simulink library "env_estimation_lib"  (R2016b)
settings: Solver=VariableStepAuto  StartTime=0.0  StopTime=10.0  RelTol=1e-3
undefined symbols (not defined in the file or in its folder): fsw_params
libraries: gs_prediction_lib x1, mag_vec_lib x1, sgp4_lib_fsw x1, sun_vector_lib x1, time_coord_rotation_lib x1
settings Model: Creator=taylorreynolds  LastModifiedBy=taylorreynolds

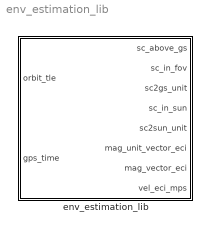
== system env_estimation_lib ==
  env_estimation_lib : Subsystem

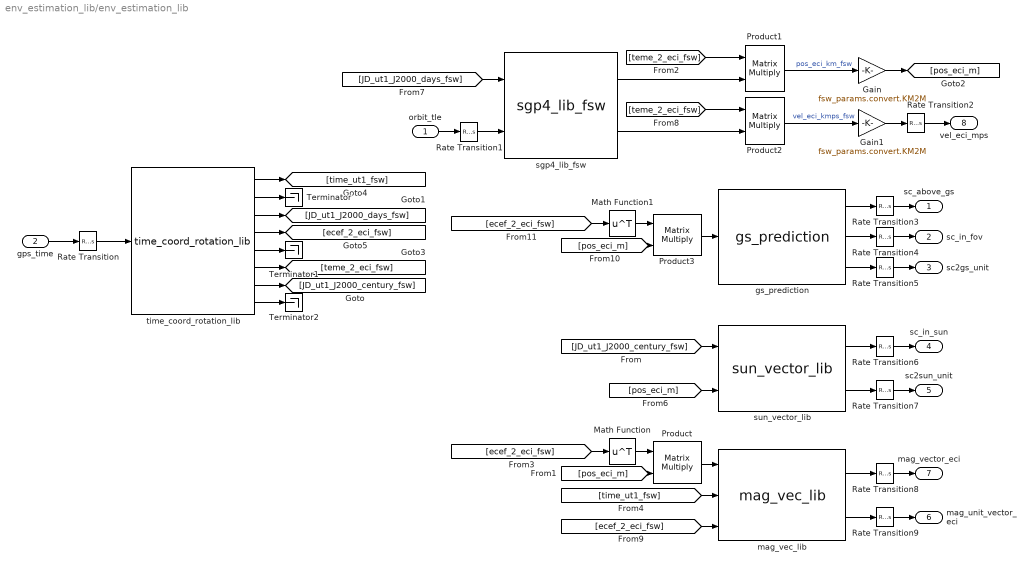
== system env_estimation_lib/env_estimation_lib ==
  orbit_tle : Inport
  gps_time : Inport  Port=2
  Gain : Gain  Gain=fsw_params.convert.KM2M
  Gain1 : Gain  Gain=fsw_params.convert.KM2M
  Math Function : Math  Operator=transpose  SaturateOnIntegerOverflow=on
  Math Function1 : Math  Operator=transpose  SaturateOnIntegerOverflow=on
  Product{,1..3} (4 alike) : Product  Multiplication=Matrix(*)
  Rate Transition : RateTransition  X0=fsw_params.env_estimation.ic.gps_time  OutPortSampleTime=fsw_params.env_estimation.sample_time_s
  Rate Transition1 : RateTransition  X0=fsw_params.env_estimation.ic.orbit_tle  OutPortSampleTime=fsw_params.env_estimation.sample_time_s
  Rate Transition{2..9} (8 alike) : RateTransition
  Terminator : Terminator
  Terminator1 : Terminator
  Terminator2 : Terminator
  gs_prediction : gs_prediction_lib/gs_prediction
  mag_vec_lib : mag_vec_lib/mag_vec_lib
  sgp4_lib_fsw : sgp4_lib_fsw/sgp4_lib_fsw
  sun_vector_lib : sun_vector_lib/sun_vector_lib
  time_coord_rotation_lib : time_coord_rotation_lib/time_coord_rotation_lib
  sc_above_gs : Outport
  sc_in_fov : Outport  Port=2
  sc2gs_unit : Outport  Port=3
  sc_in_sun : Outport  Port=4
  sc2sun_unit : Outport  Port=5
  mag_unit_vector_eci : Outport  Port=6
  mag_vector_eci : Outport  Port=7
  vel_eci_mps : Outport  Port=8
  wires:
  mag_vec_lib/2 -> Rate Transition9/1
  mag_vec_lib/1 -> Rate Transition8/1
  sun_vector_lib/2 -> Rate Transition7/1
  [teme_2_eci_fsw] -> Product1/1
  [teme_2_eci_fsw] -> Product2/1
  [ecef_2_eci_fsw] -> Math Function/1
  [JD_ut1_J2000_century_fsw] -> sun_vector_lib/1
  [JD_ut1_J2000_days_fsw] -> sgp4_lib_fsw/1
  [ecef_2_eci_fsw] -> mag_vec_lib/3
  [time_ut1_fsw] -> mag_vec_lib/2
  sun_vector_lib/1 -> Rate Transition6/1
  Product2/1 -> Gain1/1  "vel_eci_kmps_fsw"
  sgp4_lib_fsw/2 -> Product2/2
  sgp4_lib_fsw/1 -> Product1/2
  Product1/1 -> Gain/1  "pos_eci_km_fsw"
  [pos_eci_m] -> Product/2
  [pos_eci_m] -> sun_vector_lib/2
  Gain1/1 -> Rate Transition2/1
  Math Function/1 -> Product/1
  Product/1 -> mag_vec_lib/1
  Gain/1 -> [pos_eci_m]
  orbit_tle/1 -> Rate Transition1/1
  gps_time/1 -> Rate Transition/1
  time_coord_rotation_lib/2 -> Terminator/1
  time_coord_rotation_lib/4 -> [ecef_2_eci_fsw]
  time_coord_rotation_lib/6 -> [teme_2_eci_fsw]
  time_coord_rotation_lib/1 -> [time_ut1_fsw]
  time_coord_rotation_lib/3 -> [JD_ut1_J2000_days_fsw]
  time_coord_rotation_lib/7 -> [JD_ut1_J2000_century_fsw]
  gs_prediction/1 -> Rate Transition3/1
  gs_prediction/3 -> Rate Transition5/1
  gs_prediction/2 -> Rate Transition4/1
  time_coord_rotation_lib/5 -> Terminator1/1
  time_coord_rotation_lib/8 -> Terminator2/1
  Rate Transition/1 -> time_coord_rotation_lib/1
  Rate Transition1/1 -> sgp4_lib_fsw/2
  Rate Transition2/1 -> vel_eci_mps/1
  Rate Transition3/1 -> sc_above_gs/1
  Rate Transition4/1 -> sc_in_fov/1
  Rate Transition5/1 -> sc2gs_unit/1
  Rate Transition6/1 -> sc_in_sun/1
  Rate Transition7/1 -> sc2sun_unit/1
  Rate Transition8/1 -> mag_vector_eci/1
  Rate Transition9/1 -> mag_unit_vector_eci/1
  [ecef_2_eci_fsw] -> Math Function1/1
  [pos_eci_m] -> Product3/2
  Math Function1/1 -> Product3/1
  Product3/1 -> gs_prediction/1
